simulink model "frist_proble"  (R2018a)
settings: Solver=ode23tb  StartTime=0.0  StopTime=50  RelTol=1e-3
settings Model: Creator=lenovo  LastModifiedBy=lenovo

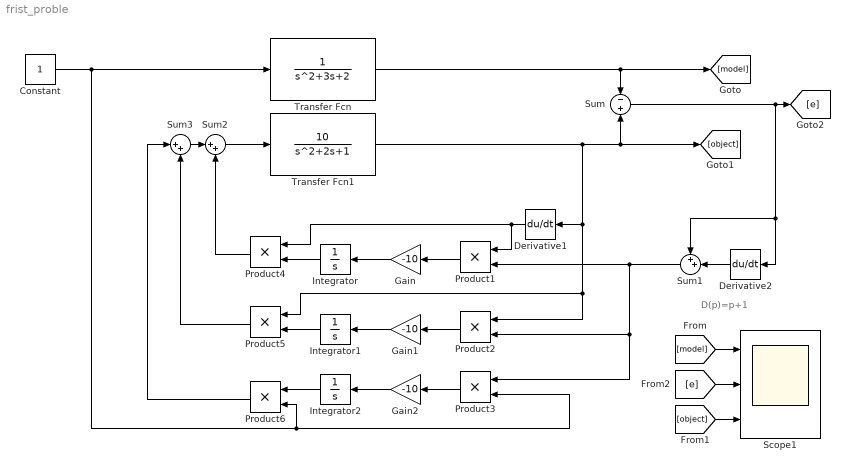
== system frist_proble ==
  note: D(p)=p+1
  Constant : Constant
  Derivative1 : Derivative
  Derivative2 : Derivative
  Gain : Gain  Gain=-10
  Gain1 : Gain  Gain=-10
  Gain2 : Gain  Gain=-10
  Integrator : Integrator
  Integrator1 : Integrator
  Integrator2 : Integrator
  Product{1..6} (6 alike) : Product
  Scope1 : Scope  NumInputPorts=3
  Sum : Sum  Inputs=-|+
  Sum1 : Sum  Inputs=++|
  Sum2 : Sum  Inputs=|++
  Sum3 : Sum  Inputs=|++
  Transfer Fcn : TransferFcn  Denominator=[1 3 2]
  Transfer Fcn1 : TransferFcn  Numerator=[10]
  wires:
  Transfer Fcn/1 -> [model], Sum/1
  Transfer Fcn1/1 -> Product5/1, Product2/1, Derivative1/1, [object], Sum/2
  Sum/1 -> [e], Sum1/1, Derivative2/1
  Derivative2/1 -> Sum1/2
  Derivative1/1 -> Product1/1, Product4/1
  Sum1/1 -> Product2/2, Product3/1, Product1/2
  Product1/1 -> Gain/1
  Product3/1 -> Gain2/1
  Product2/1 -> Gain1/1
  Gain/1 -> Integrator/1
  Gain1/1 -> Integrator1/1
  Gain2/1 -> Integrator2/1
  Integrator1/1 -> Product5/2
  Integrator2/1 -> Product6/1
  Integrator/1 -> Product4/2
  Sum2/1 -> Transfer Fcn1/1
  Product4/1 -> Sum2/2
  Sum3/1 -> Sum2/1
  Product5/1 -> Sum3/2
  Product6/1 -> Sum3/1
  [model] -> Scope1/1
  [object] -> Scope1/3
  [e] -> Scope1/2
  Constant/1 -> Transfer Fcn/1, Product6/2, Product3/2
